simulink model "Ball_Beam_testing"  (R2021b)
settings: Solver=FixedStepDiscrete  StartTime=0.0  StopTime=inf  FixedStep=0.002  RelTol=1e-3  EnableMultiTasking=on
values from neighbouring files (symbols this model uses):
  K_AMP = 1    [setup_srv02_exp04_bb01.m]
  K_BS = - L_beam / 10    [config_bb01.m]    (also in setup_srv02_exp04_bb01.m = 2 * K_BS)
  THETA_OFF = - 56.0 * K_D2R    [config_bb01.m]
  VMAX_DAC = 10    [setup_srv02_exp04_bb01.m]
undefined symbols (not defined in the file or in its folder): HIL, K_ENC, qc_get_step_size, VMAX_AMP
libraries: quarc_library x4, simulink x3, simulink_extras x1
settings Model: ExtModeTrigDuration=10000  Creator=Dell  LastModifiedBy=Dell
settings SolverCC: AlgebraicLoopSolver=TrustRegion  PositivePriorityOrder=on
settings DataIOCC: ReturnWorkspaceOutputs=off
settings DebuggingCC: SFMachineParentedDataDiag=warning  ArithmeticOperatorsInVariantConditions=warning
settings SFSimCC: SimUseLocalCustomCode=off  CustomCodeUndefinedFunction=UseInterfaceOnly
settings RTWCC: Description=QUARC Win64 Target Using Toolchain  SystemTargetFile=quarc_win64.tlc  TemplateMakefile=quarc_default_tmf  RTWUseLocalCustomCode=off  Toolchain=QUARC win64 | nmake (64-bit Windows)  BuildConfiguration=Faster Runs
settings CodeAppCC: StateflowObjectComments=on
settings STFCustomTargetCC: TargetLangStandard=C99 (ISO)  ConcurrentExecutionCompliant=on  UseToolchainInfoCompliant=on  SystemTargetFile=quarc_win64.tlc
settings GRTTargetCC: ParMdlRefBuildCompliant=off  CompOptLevelCompliant=off  CombineOutputUpdateFcns=off  MatFileLogging=off  CPPClassGenCompliant=off  GRTInterface=on  ExtMode=on  ExtModeMexFile=quarc_comm
settings ConfigComp: CovMetricSettings=dswe

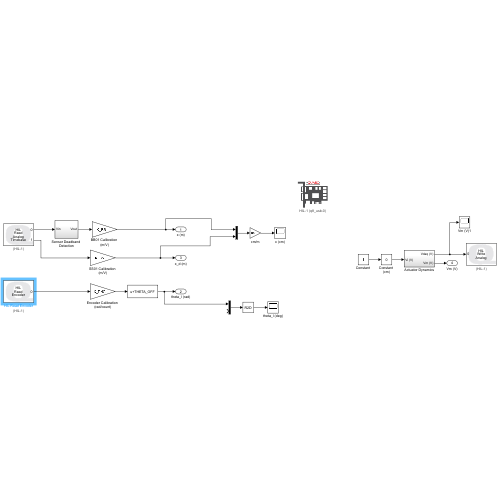
[thumbnail: Simulink's stored preview of the top-level diagram]
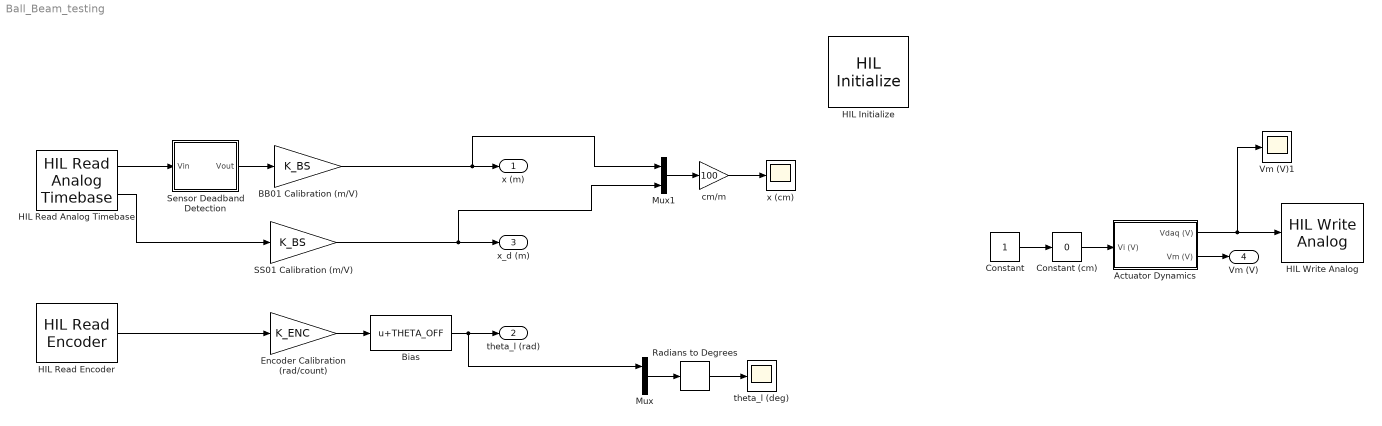
== system Ball_Beam_testing ==
  Actuator Dynamics : Subsystem
  BB01 Calibration (m/V) : Gain  Gain=K_BS  SaturateOnIntegerOverflow=on  OutDataTypeStr=Inherit: Same as input  ParamDataTypeStr=Inherit: Same as input
  Bias : Bias  Bias=THETA_OFF
  "Constant " : Constant
  Constant (cm) : simulink/Math Operations/Slider Gain  gain=0  low=-20  high=20
  Encoder Calibration (rad/count) : Gain  Gain=K_ENC  SaturateOnIntegerOverflow=on  OutDataTypeStr=Inherit: Same as input  ParamDataTypeStr=Inherit: Same as input
  HIL Initialize : quarc_library/Data Acquisition/Generic/Configuration/HIL Initialize  object_name=HIL-1  board_type=q8_usb  board_number=0  board_options=update_rate=normal  exclusive=off  active=off  hardware_clocks=[0:2]  clock_modes=[]  initial_clock_frequencies=[]  set_clock_params_at_start=off  set_clock_params_at_switch_in=off  set_clock_frequencies_at_start=off  set_clock_frequencies_at_switch_in=off  analog_input_channels=[0:7]  analog_input_configurations=[]  analog_input_maximums=10  analog_input_minimums=-10  set_analog_input_params_at_start=on  set_analog_input_params_at_switch_in=off  analog_output_channels=[0:7]  analog_output_maximums=10  analog_output_minimums=-10  initial_analog_outputs=[0]  final_analog_outputs=[0]  watchdog_analog_outputs=0  set_analog_output_params_at_start=on  set_analog_output_params_at_switch_in=off  set_analog_outputs_at_start=on  set_analog_outputs_at_switch_in=off  set_analog_outputs_at_terminate=on  set_analog_outputs_at_switch_out=off  set_analog_outputs_on_watchdog=off  digital_input_channels=[]  digital_output_channels=[0:7]  digital_output_configuration=[]  initial_digital_outputs=[0]  final_digital_outputs=[0]  watchdog_digital_outputs=[0]  set_digital_output_params_at_start=off  set_digital_output_params_at_switch_in=off  set_digital_outputs_at_start=on  set_digital_outputs_at_switch_in=off  set_digital_outputs_at_terminate=on  set_digital_outputs_at_switch_out=off  set_digital_outputs_on_watchdog=off  encoder_channels=[0:7]  quadrature=[4]  encoder_filter_frequency=[]  initial_encoder_counts=[0]  set_encoder_params_at_start=on  set_encoder_params_at_switch_in=off  set_encoder_counts_at_start=on  set_encoder_counts_at_switch_in=off  pwm_channels=[0:7]  pwm_modes=0  pwm_frequency=99.532799999999995e6/4095  pwm_configuration=[0]  pwm_alignment=[0]  pwm_polarity=[1]  pwm_leading_deadband=[0]  pwm_trailing_deadband=[0]  initial_pwm_outputs=[0]  final_pwm_outputs=[0]  watchdog_pwm_outputs=[0]  set_pwm_params_at_start=on  set_pwm_params_at_switch_in=off  set_pwm_outputs_at_start=on  set_pwm_outputs_at_switch_in=off  set_pwm_outputs_at_terminate=on  set_pwm_outputs_at_switch_out=off  set_pwm_outputs_on_watchdog=off  other_output_channels=[]  initial_other_outputs=[]  final_other_outputs=[]  watchdog_other_outputs=[]  set_other_outputs_at_start=off  set_other_outputs_at_switch_in=off  set_other_outputs_at_terminate=off  set_other_outputs_at_switch_out=off  set_other_outputs_on_watchdog=off
  HIL Read Analog Timebase : quarc_library/Data Acquisition/Generic/Timebases/HIL Read Analog Timebase  Tag=unassigned  object_name=HIL-1  channels=[0:1]  clock=0  active=on  vector_output=off  overflow_mode=Error on overflow  samples_in_buffer=max(ceil(1/qc_get_step_size), 1)
      settings: AttributesFormatString=(%<object_name>)  SourceProductName=QUARC Targets
  HIL Read Encoder : quarc_library/Data Acquisition/Generic/Immediate I//O/HIL Read Encoder  Tag=unassigned  object_name=HIL-1  channels=0  sample_time=qc_get_step_size  active=on  vector_output=off  data_type_mode=Inherit via back propagation  data_type=double
  HIL Write Analog : quarc_library/Data Acquisition/Generic/Immediate I//O/HIL Write Analog  Tag=unassigned  object_name=HIL-1  channels=0  sample_time=-1  active=off  vector_input=off
  Mux : Mux  Inputs=2
  Mux1 : Mux  Inputs=2
  Radians to Degrees : simulink_extras/Transformations/Radians to Degrees
  SS01 Calibration (m/V) : Gain  Gain=K_BS  SaturateOnIntegerOverflow=on  OutDataTypeStr=Inherit: Same as input  ParamDataTypeStr=Inherit: Same as input
  Sensor Deadband Detection : Subsystem
  Vm (V)1 : Scope
  cm/m : Gain  Gain=100
  theta_l (deg) : Scope
  x (cm) : Scope
  x (m) : Outport  InitialOutput=0
  theta_l (rad) : Outport  Port=2  InitialOutput=0
  x_d (m) : Outport  Port=3  InitialOutput=0
  Vm (V) : Outport  Port=4  InitialOutput=0
  wires:
  BB01 Calibration (m/V)/1 -> Mux1/1, x (m)/1
  Sensor Deadband Detection/1(Vout) -> BB01 Calibration (m/V)/1
  HIL Read Analog Timebase/1 -> Sensor Deadband Detection/1(Vin)
  HIL Read Analog Timebase/2 -> SS01 Calibration (m/V)/1
  HIL Read Encoder/1 -> Encoder Calibration (rad/count)/1
  SS01 Calibration (m/V)/1 -> Mux1/2, x_d (m)/1
  Bias/1 -> Mux/1, theta_l (rad)/1
  Encoder Calibration (rad/count)/1 -> Bias/1
  Actuator Dynamics/1(Vdaq (V)) -> Vm (V)1/1, HIL Write Analog/1
  Actuator Dynamics/2(Vm (V)) -> Vm (V)/1
  Constant (cm)/1 -> Actuator Dynamics/1(Vi (V))
  "Constant "/1 -> Constant (cm)/1
  Mux1/1 -> cm/m/1
  Radians to Degrees/1 -> theta_l (deg)/1
  Mux/1 -> Radians to Degrees/1
  cm/m/1 -> x (cm)/1

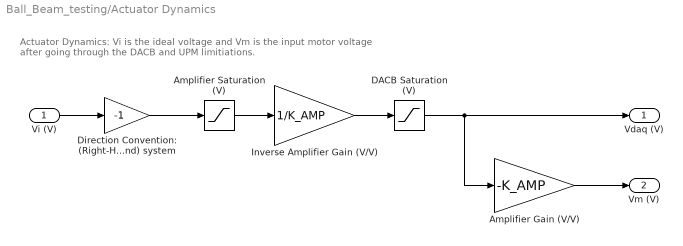
== system Ball_Beam_testing/Actuator Dynamics ==
  note: Actuator Dynamics: Vi is the ideal voltage and Vm is the
      | input motor voltage after going through the DACB and UPM limitiations.
  Vi (V) : Inport
  Amplifier Gain (V/V) : Gain  Gain=-K_AMP
  Amplifier Saturation (V) : Saturate  UpperLimit=VMAX_AMP  LowerLimit=-VMAX_AMP
  DACB Saturation (V) : Saturate  UpperLimit=VMAX_DAC  LowerLimit=-VMAX_DAC
  Direction Convention: (Right-Hand) system : Gain  Gain=-1  SaturateOnIntegerOverflow=on  OutDataTypeStr=Inherit: Same as input  ParamDataTypeStr=Inherit: Same as input
  Inverse Amplifier Gain (V/V) : Gain  Gain=1/K_AMP
  Vdaq (V) : Outport
  Vm (V) : Outport  Port=2
  wires:
  Direction Convention: (Right-Hand) system/1 -> Amplifier Saturation (V)/1
  Amplifier Gain (V/V)/1 -> Vm (V)/1
  DACB Saturation (V)/1 -> Vdaq (V)/1, Amplifier Gain (V/V)/1
  Inverse Amplifier Gain (V/V)/1 -> DACB Saturation (V)/1
  Vi (V)/1 -> Direction Convention: (Right-Hand) system/1
  Amplifier Saturation (V)/1 -> Inverse Amplifier Gain (V/V)/1

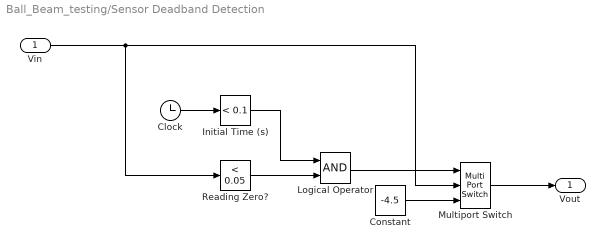
== system Ball_Beam_testing/Sensor Deadband Detection ==
  Vin : Inport
  Clock : Clock
  Constant : Constant  Value=-4.5
  Initial Time (s) : simulink/Logic and Bit Operations/Compare To Constant  relop=<  const=0.1  OutDataTypeStr=uint8  ZeroCross=off
  Logical Operator : Logic  AllPortsSameDT=off  OutDataTypeStr=boolean
  Multiport Switch : MultiPortSwitch  DataPortOrder=Zero-based contiguous  Inputs=2  zeroidx=on
  Reading Zero? : simulink/Logic and Bit Operations/Compare To Constant  relop=<  const=0.05  OutDataTypeStr=uint8  ZeroCross=off
  Vout : Outport
  wires:
  Clock/1 -> Initial Time (s)/1
  Vin/1 -> Reading Zero?/1, Multiport Switch/2
  Initial Time (s)/1 -> Logical Operator/1
  Reading Zero?/1 -> Logical Operator/2
  Logical Operator/1 -> Multiport Switch/1
  Constant/1 -> Multiport Switch/3
  Multiport Switch/1 -> Vout/1
